simulink model "MPC_DCMODEL"  (R2023b)
settings: Solver=FixedStepAuto  StartTime=0.0  StopTime=50  RelTol=1e-3
libraries: cstblocks x1, mpclib x1
settings Model: Creator=김준현  LastModifiedBy=김준현

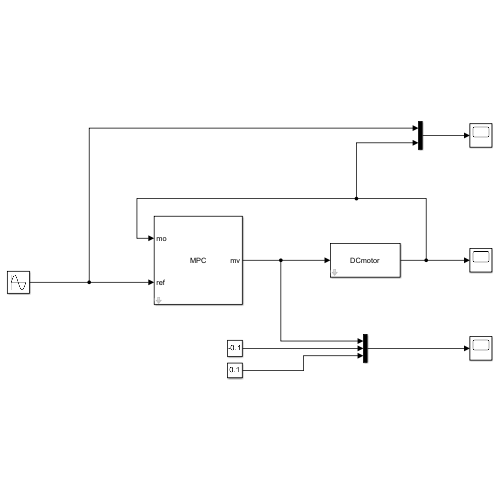
[thumbnail: Simulink's stored preview of the top-level diagram]
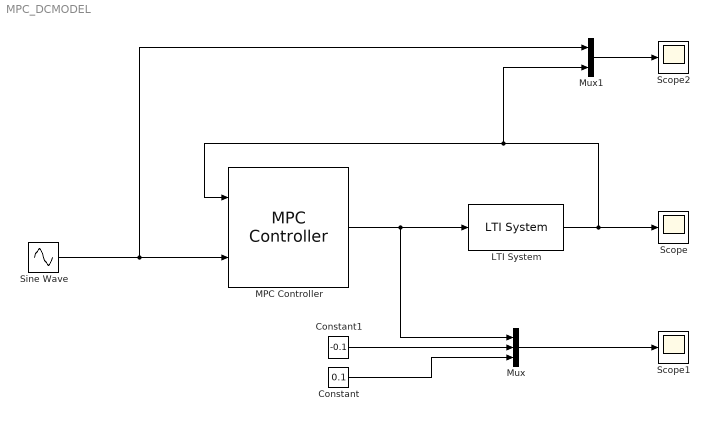
== system MPC_DCMODEL ==
  Constant : Constant  Value=0.1
  Constant1 : Constant  Value=-0.1
  LTI System : cstblocks/LTI System  sys=DCmotor  IC=[]  PadeOrder=0
  MPC Controller : mpclib/MPC Controller  SCDEnableBlockLinearizationSpecification=on  mpcobj=mpcobj  is_multiple=0  enable_value=0  return_u0=off  updateMPCinCallerWorkspace=on  md_inport=off  mv_inport=off  uref_inport=off  return_cost=off  return_mvseq=off  return_qpstatus=off  return_xseq=off  return_state=off  return_ovseq=off  state_inport=off  umin_inport=off  umax_inport=off  ymin_inport=off  ymax_inport=off  cc_inport=off  ywt_inport=off  uwt_inport=off  duwt_inport=off  rhoeps_inport=off  pm_inport=off  MaximumP=10  HorizonChoice=FixedHorizon  n_ts=0.01  n_p=10  n_mv=1  n_md=0  n_ud=0  n_mo=1  n_uo=0  BlockDataType=double  SampleTimeInherited=off  switch_inport=off
  Mux : Mux  Inputs=3
  Mux1 : Mux  Inputs=2
  Scope : Scope
  Scope1 : Scope
  Scope2 : Scope
  Sine Wave : Sin  Amplitude=pi  Frequency=0.6  SampleTime=0
  wires:
  MPC Controller/1 -> Mux/1, LTI System/1
  Sine Wave/1 -> Mux1/1, MPC Controller/2
  LTI System/1 -> Scope/1, Mux1/2, MPC Controller/1
  Mux/1 -> Scope1/1
  Constant1/1 -> Mux/2
  Constant/1 -> Mux/3
  Mux1/1 -> Scope2/1
